simulink model "lb553_rtlsdr_rx_am_fdm"  (R2018b)
settings: Solver=VariableStepAuto  StartTime=0.0  StopTime=inf  RelTol=1e-3
undefined symbols (not defined in the file): fdesignblkfcn, gcbh
libraries: dsparch4 x3, dspsnks4 x1, dspmlti4 x1, dspfdesign x1, sdrrlib x1
settings Model: Creator=Григорий Фокин  LastModifiedBy=Григорий Фокин
settings SFSimCC: SimUseLocalCustomCode=off
settings RTWCC: RTWUseLocalCustomCode=off
settings CodeAppCC: StateflowObjectComments=on

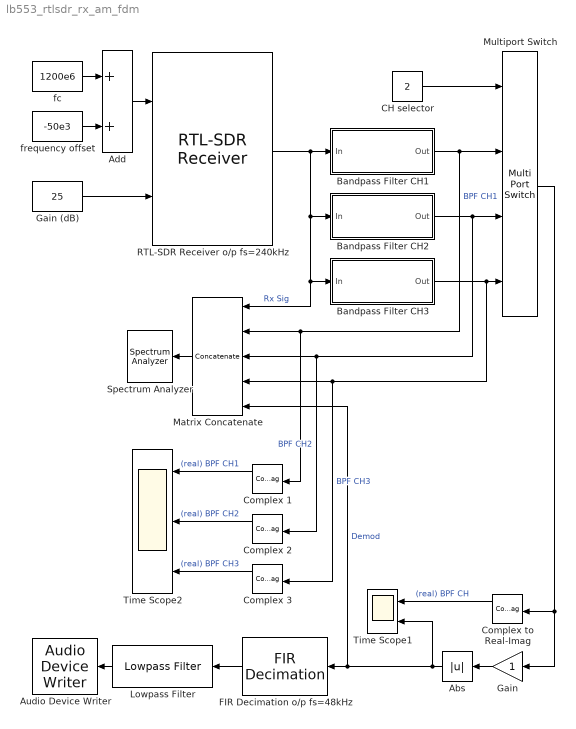
== system lb553_rtlsdr_rx_am_fdm ==
  Abs : Abs
  Add : Sum
  Audio Device Writer : dspsnks4/Audio Device Writer  Driver=DirectSound  Device=Default  InheritSampleRate=on  SampleRate=44100  BitDepth=16-bit integer  BufferSize=4096  NumBuffers=10  DefaultOutputChannelMapping=on  OutputChannelMapping=1:2  OutputNumUnderrunSamples=off  DriverIdx=1  DeviceWarnFlag=''
  Bandpass Filter CH1 : Subsystem  DialogController=fdesignblkfcn  InitFcn=fdesignblkfcn(gcbh, {'InitFcn'});  mask(Bandpass Filter){}
      mask help: Design a bandpass filter
      settings: CopyFcn=fdesignblkfcn(gcbh, {'CopyFcn'});
      mask Help: helpview(mapfilelocation('dsp'), 'dspbandpassfilter');
      mask Display: disp('Bandpass');
  Bandpass Filter CH2 : Subsystem  DialogController=fdesignblkfcn  InitFcn=fdesignblkfcn(gcbh, {'InitFcn'});  mask(Bandpass Filter){}
      mask help: Design a bandpass filter
      settings: CopyFcn=fdesignblkfcn(gcbh, {'CopyFcn'});
      mask Help: helpview(mapfilelocation('dsp'), 'dspbandpassfilter');
      mask Display: disp('Bandpass');
  Bandpass Filter CH3 : Subsystem  DialogController=fdesignblkfcn  InitFcn=fdesignblkfcn(gcbh, {'InitFcn'});  mask(Bandpass Filter){}
      mask help: Design a bandpass filter
      settings: CopyFcn=fdesignblkfcn(gcbh, {'CopyFcn'});
      mask Help: helpview(mapfilelocation('dsp'), 'dspbandpassfilter');
      mask Display: disp('Bandpass');
  CH selector : Constant  Value=2
  Complex 1 : ComplexToRealImag
  Complex 2 : ComplexToRealImag
  Complex 3 : ComplexToRealImag
  Complex to Real-Imag : ComplexToRealImag
  FIR Decimation o/p fs=48kHz : dspmlti4/FIR Decimation  FilterSource=Dialog parameters  h=firpm(100, [0 15e3 20e3 (240e3/2)]/(240e3/2), [1 1 0 0], [1 1], 20)  D=5  filtStruct=Direct form  FilterObject=FDECIM  InputProcessing=Columns as channels (frame based)  framing=Allow multirate processing  inputOffset=0  outputBufInitCond=0  roundingMode=Floor  overflowMode=off  firstCoeffDataTypeStr=Inherit: Same word length as input  firstCoeffMin=[]  firstCoeffMax=[]  firstCoeffLastDataTypeStr=Inherit: Same word length as input  outputDataTypeStr=Inherit: Same as accumulator  outputMin=[]  outputMax=[]  outputLastDataTypeStr=Inherit: Same as accumulator
  Gain : Gain
  Gain (dB) : Constant  Value=25
  Lowpass Filter : dspfdesign/Lowpass Filter  FilterType=IIR  DesignForMinimumOrder=on  FilterOrder=50  PassbandFrequency=4e3  StopbandFrequency=4.5e3  PassbandRipple=1  StopbandAttenuation=100  InheritSampleRate=off  SampleRate=48e3  SimulateUsing=Interpreted execution  roundingMode=Floor  coeffsDataTypeStr=fixdt(1,16)
  Matrix Concatenate : Concatenate  NumInputs=5  Mode=Multidimensional array  ConcatenateDimension=2
  Multiport Switch : MultiPortSwitch
  RTL-SDR Receiver o/p fs=240kHz : sdrrlib/RTL-SDR Receiver  IPAddress=0  CenterFrequencySource=Input port  CenterFrequency=102.5e6  GainSource=Input port  Gain=0  ADCRate=240e3  FrequencyCorrection=47  LostSamplesOutputPort=off  LatencyOutputPort=off  OutputDataType=single  FrameLength=4096  EnableBurstMode=off  NumFramesInBurst=20  sobjType=sdrr.internal.SDRRTLReceiverSL  dataUDPPort=-1  ctrlUDPPort=-1  subDeviceList=nosubdev  sdrBlockType=SDRBlockTypeSLT.SDRRxBlock  requester=UNUSED_BY_SFCN  sdrExecutionMode=SDRExecutionModeSLT.ExecModeHW  BypassUserLogic=off  DecimatorSelect=DDC decimator  SourceSelect=RF data  SineAmplitude=16000  EnableInternalClock=off  BypassIQBalance=off  IFBandwidth=40e6  ADCRateSource=Dialog  IntermediateFrequency=0  DecimationFactorSource=Dialog  DecimationFactor=512  RFFrequencyIsTunable=logical(1)  SampleTime=(4096)/(240e3)  IFBandwidthSource=Dialog  SineFrequency=30000  BypassDCBlockingFilter=off  IntermediateFrequencySource=Dialog  IQBalanceCoefficients=64  SkipAllHardwareResetAndInitialization=off  EnableIQCalibrationTable=on  CacheIQCalibrationTable=off  EnableOffsetTuning=off  EnableRTLAGC=off  EnableTestMode=off  EnableTunerAGC=off  FrequencyCorrectionSource=Dialog  NumMLBuffers=128  NumUSBBuffers=16  RTLCrystalFrequency=28800000  TunerCrystalFrequency=28800000
      settings: SourceProductName=Communications System Toolbox Support Package for RTL-SDR Radio  SourceProductBaseCode=RTLSDR
  Spectrum Analyzer : SpectrumAnalyzer
  Time Scope1 : Scope  NumInputPorts=2
  Time Scope2 : Scope  NumInputPorts=3
  fc : Constant  Value=1200e6
  frequency offset : Constant  Value=-50e3
  wires:
  Add/1 -> RTL-SDR Receiver o/p fs=240kHz/1
  fc/1 -> Add/1
  frequency offset/1 -> Add/2
  Gain (dB)/1 -> RTL-SDR Receiver o/p fs=240kHz/2
  RTL-SDR Receiver o/p fs=240kHz/1 -> Matrix Concatenate/1, Bandpass Filter CH3/1(In), Bandpass Filter CH2/1(In), Bandpass Filter CH1/1(In)  "Rx Sig"
  CH selector/1 -> Multiport Switch/1
  Bandpass Filter CH1/1(Out) -> Complex 1/1, Matrix Concatenate/2, Multiport Switch/2  "BPF CH1"
  Bandpass Filter CH2/1(Out) -> Complex 2/1, Matrix Concatenate/3, Multiport Switch/3  "BPF CH2"
  Bandpass Filter CH3/1(Out) -> Complex 3/1, Matrix Concatenate/4, Multiport Switch/4  "BPF CH3"
  Multiport Switch/1 -> Complex to Real-Imag/1, Gain/1
  Gain/1 -> Abs/1
  Abs/1 -> Matrix Concatenate/5, FIR Decimation o/p fs=48kHz/1, Time Scope1/2  "Demod"
  FIR Decimation o/p fs=48kHz/1 -> Lowpass Filter/1
  Lowpass Filter/1 -> Audio Device Writer/1
  Matrix Concatenate/1 -> Spectrum Analyzer/1
  Complex to Real-Imag/1 -> Time Scope1/1  "(real) BPF CH"
  Complex 1/1 -> Time Scope2/1  "(real) BPF CH1"
  Complex 2/1 -> Time Scope2/2  "(real) BPF CH2"
  Complex 3/1 -> Time Scope2/3  "(real) BPF CH3"

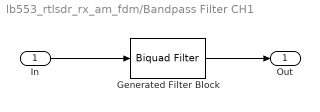
== system lb553_rtlsdr_rx_am_fdm/Bandpass Filter CH1 ==
  In : Inport
  Generated Filter Block : dsparch4/Biquad Filter  Tag=BlockMethodSubSystem  FilterSource=Dialog parameters  CoeffSource=Specify via dialog  FilterObject=BQF  IIRFiltStruct=Direct form II  BiQuadCoeffs=[0.67725504711171325 -0.63458623437762918 0.70569823443816759 1 -0.68790893342333459 0.95122225152324946;0.76912318957175352 -0.10503304004140397 0.75300830902983529 1 -0.31748660626909891 0.94907304896556866;0.87477423956609845 -1.1975807514346279 0.41753394632541252 1 -0.49406504940848572 0.89541618790484334;-0.0099984491901301664 -0.0054378645625562695 -0.00071914015742973131 1 -0.2199444385652696 0.001741879196407548;1.2169119181963859 -0.93350870960493404 1.2166167073062797 1 -0.74304185104344955 0.9944853261285258;2 -0.51811163988052578 1.9995757578025131 1 -0.28194844272200936 0.99446165339494519;0.61779951634553276 -0.64291941769811833 0.26128725510466211 1 -0.60815197140679966 0.91558904093798277;0.034237823506261256 -0.0027884025484853584 0.00016769300714795474 1 -0.38453782819370719 0.91150339975020866;0.93259767836924201 -0.73412112428315779 0.93243700672985008 1 -0.72765318850537697 0.97889590780235269;2 -0.47619246180128105 1.9980358564719718 1 -0.28997318981062714 0.97851123594504019]  ScaleValues=[0.045643880161879133;1;1;1;1;1;1;1;1;1;10.298014278585658]  IC=0  ICnum=0  ICden=0  a0Flag=Warning  optimizeScaleValues=off  ScaleValueMode=Specify via input port (g)  InputProcessing=Columns as channels (frame based)  roundingMode=Floor  overflowMode=off  scaleValueFracLength=14  denProdOutputFracLength=30  denAccumFracLength=30  secondMemoryFracLength=15
      settings: SourceProductName=DSP System Toolbox
  Out : Outport
  wires:
  In/1 -> Generated Filter Block/1
  Generated Filter Block/1 -> Out/1

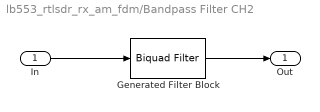
== system lb553_rtlsdr_rx_am_fdm/Bandpass Filter CH2 ==
  In : Inport
  Generated Filter Block : dsparch4/Biquad Filter  Tag=BlockMethodSubSystem  FilterSource=Dialog parameters  CoeffSource=Specify via dialog  FilterObject=BQF  IIRFiltStruct=Direct form II  BiQuadCoeffs=[0.66152503103721549 -0.27527902054278863 0.64732566253185497 1 -0.20133865126739836 0.9588779662340825;0.77534026721793858 0.28633240403099786 0.75302305916323087 1 0.20127857789942211 0.958317376045979;0.1583774515563304 0.015471428449544855 0.0010593621464747077 1 -0.054672447558420351 0.90396091523826394;0.018068618698837378 0.00048970837663502454 2.1493938425407724e-05 1 0.051877867134379085 0.90305357870725111;1.2414148449034801 -0.32620453745389455 1.241372431485968 1 -0.23880467262613786 0.99498496646894019;2 0.52555948795200391 1.9999636648018655 1 0.23883048071077961 0.99498152885433144;0.75085259726786435 -0.45727914677615616 0.7298698728890789 1 -0.1447276981533081 0.92848952219889458;0.038092822325368959 0.035666985507320267 0.036829375679378155 1 0.14363520470362284 0.92710571866366787;0.88289255317355553 -0.24822776297737748 0.88209402053737951 1 -0.22861707262432496 0.98150146687754047;1.9999999999999998 0.56040592978426329 1.9949736003473875 1 0.22866633795811103 0.98141882779970846]  ScaleValues=[0.040905194732946029;1;1;1;1;1;1;1;1;1;11.109235270428163]  IC=0  ICnum=0  ICden=0  a0Flag=Warning  optimizeScaleValues=off  ScaleValueMode=Specify via input port (g)  InputProcessing=Columns as channels (frame based)  roundingMode=Floor  overflowMode=off  scaleValueFracLength=14  denProdOutputFracLength=30  denAccumFracLength=30  secondMemoryFracLength=15
      settings: SourceProductName=DSP System Toolbox
  Out : Outport
  wires:
  Generated Filter Block/1 -> Out/1
  In/1 -> Generated Filter Block/1

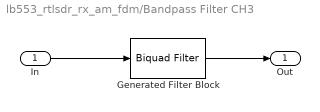
== system lb553_rtlsdr_rx_am_fdm/Bandpass Filter CH3 ==
  In : Inport
  Generated Filter Block : dsparch4/Biquad Filter  Tag=BlockMethodSubSystem  FilterSource=Dialog parameters  CoeffSource=Specify via dialog  FilterObject=BQF  IIRFiltStruct=Direct form II  BiQuadCoeffs=[0.66523374352053077 -0.9163494089443418 0.61344965733873758 1 -1.1383127525849286 0.95333829204222909;0.37868582367945297 -0.13161618638648059 0.35433876751253812 1 -0.80397629534196824 0.95132331725279107;0.21851967019578275 -0.18555481534182797 0.038942783341401992 1 -0.95958201198723903 0.89328180813032687;0.023915938476271638 -0.040572779541590012 0.017182138443266635 1 -0.84799671673304 0.83837189040549687;0.4112386643347945 -0.50132606550921299 0.41119595795835745 1 -1.1967189778645153 0.99457760357656566;2 -1.5269608539238377 1.9998884500895073 1 -0.78349057238092112 0.99454600746697708;1.2034636095621696 -0.37390071618136322 1.1906699030456858 1 -1.0637858285094457 0.92018169890848034;0.026572935495340556 0.0068920581816241675 0.0058303208618908017 1 -0.84784280079060625 0.90890233676847265;1.0114677957339449 -1.2506228156108723 1.0106286935217732 1 -1.1792009890213526 0.97939639439508119;2 -1.4855026747217364 1.9987059500569604 1 -0.78691199160225689 0.97910874747676213]  ScaleValues=[0.03791444614236613;1;1;1;1;1;1;1;1;1;10.789517859313694]  IC=0  ICnum=0  ICden=0  a0Flag=Warning  optimizeScaleValues=off  ScaleValueMode=Specify via input port (g)  InputProcessing=Columns as channels (frame based)  roundingMode=Floor  overflowMode=off  scaleValueFracLength=14  denProdOutputFracLength=30  denAccumFracLength=30  secondMemoryFracLength=15
      settings: SourceProductName=DSP System Toolbox
  Out : Outport
  wires:
  In/1 -> Generated Filter Block/1
  Generated Filter Block/1 -> Out/1
